simulink model "Hospital"  (R2023b)
settings: Solver=VariableStepAuto  StartTime=0.0  StopTime=10.0  RelTol=1e-3
(part 2 of 2)

== matlab function Hospital/media ==
  data: u input; y output
function y = media(u)

y = mean(u);

== matlab function Hospital/media2 ==
  data: u input; y output
function y = media(u)

y = mean(u);

== matlab function Hospital/media3 ==
  data: u input; y output
function y = media(u)

y = mean(u);

== matlab function Hospital/media4 ==
  data: u input; y output
function y = media(u)

y = mean(u);

== matlab function Hospital/media1 ==
  data: u input; y output
function y = media(u)

y = mean(u);
